simulink model "gps_tracking_onlydll_hwc_2"  (R2018a)
settings: Solver=VariableStepAuto  StartTime=0.0  StopTime=10*16368/16367600  RelTol=1e-3
libraries: xbsIndex_r4 x101, dspsrcs4 x1
settings Model: Creator=zhati  LastModifiedBy=Doc_v
settings CodeAppCC: StateflowObjectComments=on
settings SimscapeCC: SimscapeNormalizeSystem=off

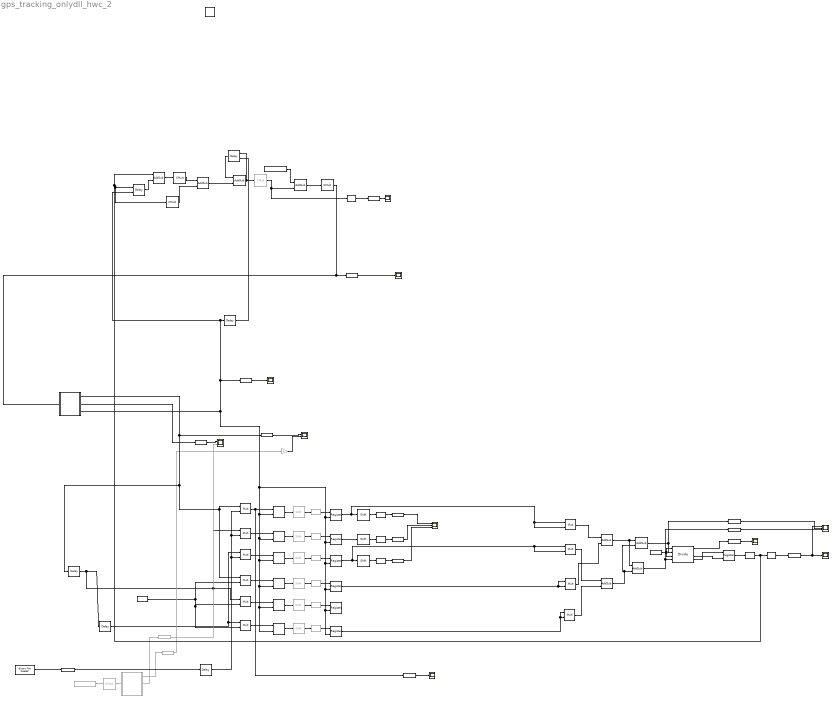
== system gps_tracking_onlydll_hwc_2 ==
  note: Subsystem1
  note: Subsystem
  note: Subsystem1
  " I_P_Out" : xbsIndex_r4/Gateway Out  inherit_from_input=on  hdl_port=on  rows=1  columns=1  UseAsDAC=off  DACChannel='1'  interface=None  automatic_assignment=on  address_offset=hex2dec('00')  intf_name=''  intf_description=''  timing_constraint=None  locs_specified=off  LOCs={}  io_standard={}  block_type=gatewayout
  " System Generator" : xbsIndex_r4/ System Generator  Tag=genX  xilinxfamily=kintex7  part=xc7k325t  speed=-2  package=ffg900  synthesis_tool=Vivado  clock_wrapper=Clock Enables  directory=./gps_tracking_onlydll_hwc2  proj_type=Vivado  Synth_file=Vivado Synthesis Defaults  Impl_file=Vivado Implementation Defaults  testbench=on  simulink_period=1/16367600  sysclk_period=10  dcm_input_clock_period=10  incr_netlist=off  trim_vbits=Everywhere in SubSystem  dbl_ovrd=According to Block Masks  core_generation=According to Block Masks  run_coregen=off  deprecated_control=off  eval_field=0  block_type=sysgen
  Accumulator{,1..5} (6 alike) : xbsIndex_r4/Accumulator  operation=Add  n_bits=20  overflow=Wrap  scale=1  rst=on  hasbypass=off  infoeditControl=reset for floating point data type must be asserted for a minimum of 2 cycles  en=off  latency=1  msb_inp=100  msb=100  lsb=-100  use_behavioral_HDL=on  implementation=Fabric  dbl_ovrd=off  block_type=accum
  AddSub10 : xbsIndex_r4/AddSub  mode=Addition  use_carryin=off  use_carryout=off  en=off  latency=1  precision=User Defined  arith_type="Signed  (2's comp)"  n_bits=35  bin_pt=0  quantization=Truncate  overflow=Flag as error  use_behavioral_HDL=off  hw_selection=Fabric  pipelined=off  dbl_ovrd=off  block_type=addsub
  AddSub11 : xbsIndex_r4/AddSub  mode=Subtraction  use_carryin=off  use_carryout=off  en=off  latency=1  precision=User Defined  arith_type="Signed  (2's comp)"  n_bits=35  bin_pt=0  quantization=Truncate  overflow=Flag as error  use_behavioral_HDL=off  hw_selection=Fabric  pipelined=off  dbl_ovrd=off  block_type=addsub
  AddSub{5,7,9,12} (4 alike) : xbsIndex_r4/AddSub  mode=Addition  use_carryin=off  use_carryout=off  en=off  latency=1  precision=Full  arith_type="Signed  (2's comp)"  n_bits=16  bin_pt=15  quantization=Truncate  overflow=Wrap  use_behavioral_HDL=off  hw_selection=Fabric  pipelined=off  dbl_ovrd=off  block_type=addsub
  AddSub2 : xbsIndex_r4/AddSub  mode=Subtraction  use_carryin=off  use_carryout=off  en=off  latency=1  precision=Full  arith_type="Signed  (2's comp)"  n_bits=16  bin_pt=15  quantization=Truncate  overflow=Wrap  use_behavioral_HDL=off  hw_selection=Fabric  pipelined=off  dbl_ovrd=off  block_type=addsub
  AddSub6 : xbsIndex_r4/AddSub  mode=Addition  use_carryin=off  use_carryout=off  en=off  latency=1  precision=User Defined  arith_type="Signed  (2's comp)"  n_bits=32  bin_pt=15  quantization=Truncate  overflow=Flag as error  use_behavioral_HDL=off  hw_selection=Fabric  pipelined=off  dbl_ovrd=off  block_type=addsub
  Binary File Reader : dspsrcs4/Binary File Reader  Filename=E:\sysgen_workspace\myGNSSdata_BB.bin  HeaderStructure=struct([])  DataType=int8  SamplesPerFrame=1  IsDataComplex=off  NumChannels=1  OutputEOF=off  SampleTime=1/16367600  SimulateUsing=Code generation
      settings: SourceProductName=DSP System Toolbox  SourceProductBaseCode=DS
  Constant : xbsIndex_r4/Constant  const=0  gui_display_data_type=Fixed-point  arith_type=Signed (2's comp)  n_bits=4  bin_pt=3  preci_type=Single  exp_width=8  frac_width=24  explicit_period=on  period=1/16367600  equ=P=C  opselect=C  inp2=PCIN>>17  opr=+  inp1=P  carry=CIN  dbl_ovrd=off  block_type=constant
  Constant1 : xbsIndex_r4/Constant  const=1.0  gui_display_data_type=Boolean  arith_type=Boolean  n_bits=16  bin_pt=14  preci_type=Single  exp_width=8  frac_width=24  explicit_period=off  period=1  equ=P=C  opselect=C  inp2=PCIN>>17  opr=+  inp1=P  carry=CIN  dbl_ovrd=off  block_type=constant
  Convert : xbsIndex_r4/Convert  gui_display_data_type=Fixed-point  arith_type="Signed  (2's comp)"  n_bits=16  bin_pt=0  float_type=Single  exp_bits=8  fraction_bits=24  quantization=Truncate  overflow=Saturate  en=off  latency=1  pipeline=off  dbl_ovrd=off  block_type=convert
  Convert{1..6} (6 alike) : xbsIndex_r4/Convert  Commented=through  gui_display_data_type=Fixed-point  arith_type="Signed  (2's comp)"  n_bits=26  bin_pt=26  float_type=Single  exp_bits=8  fraction_bits=24  quantization=Truncate  overflow=Flag as error  en=off  latency=1  pipeline=off  dbl_ovrd=off  block_type=convert
  Convert10 : xbsIndex_r4/Convert  gui_display_data_type=Fixed-point  arith_type="Signed  (2's comp)"  n_bits=8  bin_pt=4  float_type=Single  exp_bits=8  fraction_bits=24  quantization=Truncate  overflow=Saturate  en=off  latency=1  pipeline=off  dbl_ovrd=off  block_type=convert
  Convert11 : xbsIndex_r4/Convert  gui_display_data_type=Fixed-point  arith_type="Signed  (2's comp)"  n_bits=8  bin_pt=7  float_type=Single  exp_bits=8  fraction_bits=24  quantization=Truncate  overflow=Saturate  en=off  latency=1  pipeline=off  dbl_ovrd=off  block_type=convert
  Convert7 : xbsIndex_r4/Convert  gui_display_data_type=Fixed-point  arith_type="Signed  (2's comp)"  n_bits=8  bin_pt=0  float_type=Single  exp_bits=8  fraction_bits=24  quantization=Truncate  overflow=Saturate  en=off  latency=1  pipeline=off  dbl_ovrd=off  block_type=convert
  Convert8 : xbsIndex_r4/Convert  gui_display_data_type=Fixed-point  arith_type="Signed  (2's comp)"  n_bits=8  bin_pt=0  float_type=Single  exp_bits=8  fraction_bits=24  quantization=Truncate  overflow=Saturate  en=off  latency=1  pipeline=off  dbl_ovrd=off  block_type=convert
  Convert9 : xbsIndex_r4/Convert  gui_display_data_type=Fixed-point  arith_type="Signed  (2's comp)"  n_bits=16  bin_pt=14  float_type=Single  exp_bits=8  fraction_bits=24  quantization=Truncate  overflow=Saturate  en=off  latency=1  pipeline=off  dbl_ovrd=off  block_type=convert
  D1 : xbsIndex_r4/CMult  const=5.297297  gui_display_data_type=Fixed-point  const_n_bits=20  const_bin_pt=15  float_type=Single  exp_bits=8  fraction_bits=24  en=off  latency=1  precision=Full  arith_type="Signed  (2's comp)"  n_bits=16  bin_pt=14  quantization=Truncate  overflow=Wrap  use_behavioral_HDL=off  mem_type=Distributed RAM  pipeline=off  dbl_ovrd=off  block_type=cmult
  D2 : xbsIndex_r4/CMult  const=1/16367600  gui_display_data_type=Fixed-point  const_n_bits=48  const_bin_pt=48  float_type=Single  exp_bits=8  fraction_bits=24  en=off  latency=1  precision=User Defined  arith_type="Signed  (2's comp)"  n_bits=32  bin_pt=32  quantization=Truncate  overflow=Flag as error  use_behavioral_HDL=off  mem_type=Distributed RAM  pipeline=off  dbl_ovrd=off  block_type=cmult
  D3 : xbsIndex_r4/CMult  Commented=through  const=10  gui_display_data_type=Fixed-point  const_n_bits=8  const_bin_pt=0  float_type=Single  exp_bits=8  fraction_bits=24  en=off  latency=1  precision=User Defined  arith_type="Signed  (2's comp)"  n_bits=26  bin_pt=16  quantization=Truncate  overflow=Flag as error  use_behavioral_HDL=off  mem_type=Distributed RAM  pipeline=off  dbl_ovrd=off  block_type=cmult
  D4 : xbsIndex_r4/CMult  Commented=on  const=1/16367600  gui_display_data_type=Fixed-point  const_n_bits=48  const_bin_pt=48  float_type=Single  exp_bits=8  fraction_bits=24  en=off  latency=1  precision=User Defined  arith_type="Signed  (2's comp)"  n_bits=26  bin_pt=22  quantization=Truncate  overflow=Flag as error  use_behavioral_HDL=off  mem_type=Distributed RAM  pipeline=off  dbl_ovrd=off  block_type=cmult
  DLLFilteredOut : xbsIndex_r4/Gateway Out  inherit_from_input=off  hdl_port=on  rows=1  columns=1  UseAsDAC=off  DACChannel='1'  interface=None  automatic_assignment=on  address_offset=hex2dec('00')  intf_name=''  intf_description=''  timing_constraint=None  locs_specified=off  LOCs={}  io_standard={}  block_type=gatewayout
  DLLRawDiscriminatorOut : xbsIndex_r4/Gateway Out  inherit_from_input=on  hdl_port=on  rows=1  columns=1  UseAsDAC=off  DACChannel='1'  interface=None  automatic_assignment=on  address_offset=hex2dec('00')  intf_name=''  intf_description=''  timing_constraint=None  locs_specified=off  LOCs={}  io_standard={}  block_type=gatewayout
  Delay2 : xbsIndex_r4/Delay  rst=off  infoeditControl=Selection of Reset will increase slice count due to use of real FFs and instead of SRLs  en=off  latency=28  reg_retiming=off  dbl_ovrd=off  block_type=delay
  Delay4 : xbsIndex_r4/Delay  rst=off  infoeditControl=Selection of Reset will increase slice count due to use of real FFs and instead of SRLs  en=off  latency=8  reg_retiming=off  dbl_ovrd=off  block_type=delay
  Delay5 : xbsIndex_r4/Delay  rst=off  infoeditControl=Selection of Reset will increase slice count due to use of real FFs and instead of SRLs  en=on  latency=1  reg_retiming=off  dbl_ovrd=off  block_type=delay
  Delay6 : xbsIndex_r4/Delay  rst=off  infoeditControl=Selection of Reset will increase slice count due to use of real FFs and instead of SRLs  en=off  latency=8  reg_retiming=off  dbl_ovrd=off  block_type=delay
  Delay7 : xbsIndex_r4/Delay  rst=off  infoeditControl=Selection of Reset will increase slice count due to use of real FFs and instead of SRLs  en=on  latency=1  reg_retiming=off  dbl_ovrd=off  block_type=delay
  Delay8 : xbsIndex_r4/Delay  rst=off  infoeditControl=Selection of Reset will increase slice count due to use of real FFs and instead of SRLs  en=off  latency=3  reg_retiming=off  dbl_ovrd=off  block_type=delay
  Divide : xbsIndex_r4/Divide  flow_control=Blocking  axi_optimize_goal=Resources  algorithm_type=High_Radix  infoedit1=Specify output fraction-width for Fixed-point division.  fractional_width=14  infoedit2=Specify latency for Floating-point division.  latency=1  rate=1  has_a_tlast=off  has_a_tuser=off  has_b_tlast=off  has_b_tuser=off  en=off  has_result_tready=off  result_tlast_behv=Pass_A_TLAST  has_underflow=off  has_overflow=off  has_invalid_op=off  has_divide_by_zero=off  fpo_op_type=mergeddivide  block_type=divide
      settings: infoedit=Blocking: Wait for data on all inputs, allow back-pressure.<br>NonBlocking: operate every cycle in which all inputs are valid, no back-pressure.
  E_I : xbsIndex_r4/Mult  precision=Full  arith_type="Signed  (2's comp)"  n_bits=16  bin_pt=14  quantization=Truncate  overflow=Wrap  en=off  latency=1  use_behavioral_HDL=off  opt=Speed  use_embedded=on  optimum_pipeline=off  pipeline=on  dbl_ovrd=off  use_rpm=on  placement_style=Triangular  block_type=mult
  E_Q : xbsIndex_r4/Mult  precision=Full  arith_type="Signed  (2's comp)"  n_bits=16  bin_pt=14  quantization=Truncate  overflow=Wrap  en=off  latency=1  use_behavioral_HDL=off  opt=Speed  use_embedded=on  optimum_pipeline=off  pipeline=on  dbl_ovrd=off  use_rpm=on  placement_style=Triangular  block_type=mult
  E_mult : xbsIndex_r4/Mult  precision=Full  arith_type="Signed  (2's comp)"  n_bits=16  bin_pt=14  quantization=Truncate  overflow=Wrap  en=off  latency=1  use_behavioral_HDL=off  opt=Speed  use_embedded=on  optimum_pipeline=off  pipeline=on  dbl_ovrd=off  use_rpm=on  placement_style=Triangular  block_type=mult
  E_mult1 : xbsIndex_r4/Mult  precision=Full  arith_type="Signed  (2's comp)"  n_bits=16  bin_pt=14  quantization=Truncate  overflow=Wrap  en=off  latency=1  use_behavioral_HDL=off  opt=Speed  use_embedded=on  optimum_pipeline=off  pipeline=on  dbl_ovrd=off  use_rpm=on  placement_style=Triangular  block_type=mult
  F1 : xbsIndex_r4/Constant  const=1023000  gui_display_data_type=Fixed-point  arith_type=Signed (2's comp)  n_bits=32  bin_pt=8  preci_type=Single  exp_width=8  frac_width=24  explicit_period=on  period=1/16367600  equ=P=C  opselect=C  inp2=PCIN>>17  opr=+  inp1=P  carry=CIN  dbl_ovrd=off  block_type=constant
  F2 : xbsIndex_r4/Constant  Commented=on  const=1023000  gui_display_data_type=Fixed-point  arith_type=Signed (2's comp)  n_bits=32  bin_pt=8  preci_type=Single  exp_width=8  frac_width=24  explicit_period=on  period=1/16367600  equ=P=C  opselect=C  inp2=PCIN>>17  opr=+  inp1=P  carry=CIN  dbl_ovrd=off  block_type=constant
  Gain1 : Gain  Commented=through  Gain=5
  Gateway Out{3,6..8} (4 alike) : xbsIndex_r4/Gateway Out  inherit_from_input=off  hdl_port=off  rows=1  columns=1  UseAsDAC=off  DACChannel='1'  interface=None  automatic_assignment=on  address_offset=hex2dec('00')  intf_name=''  intf_description=''  timing_constraint=None  locs_specified=off  LOCs={}  io_standard={}  block_type=gatewayout
  Gateway Out4 : xbsIndex_r4/Gateway Out  Commented=on  inherit_from_input=off  hdl_port=off  rows=1  columns=1  UseAsDAC=off  DACChannel='1'  interface=None  automatic_assignment=on  address_offset=hex2dec('00')  intf_name=''  intf_description=''  timing_constraint=None  locs_specified=off  LOCs={}  io_standard={}  block_type=gatewayout
  Gateway Out_A : xbsIndex_r4/Gateway Out  inherit_from_input=off  hdl_port=off  rows=1  columns=1  UseAsDAC=off  DACChannel='1'  interface=None  automatic_assignment=on  address_offset=hex2dec('00')  intf_name=''  intf_description=''  timing_constraint=None  locs_specified=off  LOCs={}  io_standard={}  block_type=gatewayout
  Gateway Out_B : xbsIndex_r4/Gateway Out  inherit_from_input=off  hdl_port=off  rows=1  columns=1  UseAsDAC=off  DACChannel='1'  interface=None  automatic_assignment=on  address_offset=hex2dec('00')  intf_name=''  intf_description=''  timing_constraint=None  locs_specified=off  LOCs={}  io_standard={}  block_type=gatewayout
  I2 : xbsIndex_r4/CMult  const=0.014317  gui_display_data_type=Fixed-point  const_n_bits=20  const_bin_pt=15  float_type=Single  exp_bits=8  fraction_bits=24  en=off  latency=2  precision=Full  arith_type="Signed  (2's comp)"  n_bits=16  bin_pt=14  quantization=Truncate  overflow=Wrap  use_behavioral_HDL=off  mem_type=Distributed RAM  pipeline=off  dbl_ovrd=off  block_type=cmult
  IF In : xbsIndex_r4/Gateway In  gui_display_data_type=Fixed-point  arith_type="Signed  (2's comp)"  n_bits=3  bin_pt=0  preci_type=Single  exp_width=8  frac_width=24  rows=1  columns=1  quantization="Round  (unbiased: +/- Inf)"  overflow=Flag as error  period=1/16367600  UseAsADC=off  ADCChannel='1'  interface=None  automatic_assignment=on  address_offset=hex2dec('00')  intf_name=''  intf_description=''  default_value=0  timing_constraint=None  locs_specified=off  LOCs={}  io_standard={}  inherit_from_input=off  hdl_port=on  dbl_ovrd=off  block_type=gatewayin
  IF Out : xbsIndex_r4/Gateway Out  Commented=on  inherit_from_input=off  hdl_port=off  rows=1  columns=1  UseAsDAC=off  DACChannel='1'  interface=None  automatic_assignment=on  address_offset=hex2dec('00')  intf_name=''  intf_description=''  timing_constraint=None  locs_specified=off  LOCs={}  io_standard={}  block_type=gatewayout
  I_E_Out : xbsIndex_r4/Gateway Out  inherit_from_input=on  hdl_port=on  rows=1  columns=1  UseAsDAC=off  DACChannel='1'  interface=None  automatic_assignment=on  address_offset=hex2dec('00')  intf_name=''  intf_description=''  timing_constraint=None  locs_specified=off  LOCs={}  io_standard={}  block_type=gatewayout
  I_L_Out : xbsIndex_r4/Gateway Out  inherit_from_input=on  hdl_port=on  rows=1  columns=1  UseAsDAC=off  DACChannel='1'  interface=None  automatic_assignment=on  address_offset=hex2dec('00')  intf_name=''  intf_description=''  timing_constraint=None  locs_specified=off  LOCs={}  io_standard={}  block_type=gatewayout
  L_I : xbsIndex_r4/Mult  precision=Full  arith_type="Signed  (2's comp)"  n_bits=16  bin_pt=14  quantization=Truncate  overflow=Wrap  en=off  latency=1  use_behavioral_HDL=off  opt=Speed  use_embedded=on  optimum_pipeline=off  pipeline=on  dbl_ovrd=off  use_rpm=on  placement_style=Triangular  block_type=mult
  L_Q : xbsIndex_r4/Mult  precision=Full  arith_type="Signed  (2's comp)"  n_bits=16  bin_pt=14  quantization=Truncate  overflow=Wrap  en=off  latency=1  use_behavioral_HDL=off  opt=Speed  use_embedded=on  optimum_pipeline=off  pipeline=on  dbl_ovrd=off  use_rpm=on  placement_style=Triangular  block_type=mult
  Multi Out : xbsIndex_r4/Gateway Out  inherit_from_input=off  hdl_port=off  rows=1  columns=1  UseAsDAC=off  DACChannel='1'  interface=None  automatic_assignment=on  address_offset=hex2dec('00')  intf_name=''  intf_description=''  timing_constraint=None  locs_specified=off  LOCs={}  io_standard={}  block_type=gatewayout
  PNGen Out : xbsIndex_r4/Gateway Out  inherit_from_input=off  hdl_port=off  rows=1  columns=1  UseAsDAC=off  DACChannel='1'  interface=None  automatic_assignment=on  address_offset=hex2dec('00')  intf_name=''  intf_description=''  timing_constraint=None  locs_specified=off  LOCs={}  io_standard={}  block_type=gatewayout
  Register{1..7} (7 alike) : xbsIndex_r4/Register  init=0  rst=off  en=on  dbl_ovrd=off  block_type=register
  Scope : Scope
  Scope1 : Scope
  Scope2_en : Scope
  Scope6 : Scope  NumInputPorts=2
  Scope_CACode : Scope  NumInputPorts=2
  Scope_CodeFreq : Scope
  Scope_DLLDiscriminator : Scope  NumInputPorts=3
  Scope_I_ELP : Scope  NumInputPorts=3
  Scope_MultiResult : Scope
  Shift{,1..5} (6 alike) : xbsIndex_r4/Shift  Commented=through  shift_dir=Right  shift_bits=16  en=off  latency=1  precision=Full  arith_type="Signed  (2's comp)"  n_bits=16  bin_pt=14  quantization=Truncate  overflow=Wrap  dbl_ovrd=off  block_type=shift
  Shift6 : xbsIndex_r4/Shift  shift_dir=Right  shift_bits=8  en=off  latency=1  precision=Full  arith_type="Signed  (2's comp)"  n_bits=16  bin_pt=14  quantization=Truncate  overflow=Wrap  dbl_ovrd=off  block_type=shift
  Shift7 : xbsIndex_r4/Shift  shift_dir=Right  shift_bits=8  en=off  latency=1  precision=Full  arith_type="Signed  (2's comp)"  n_bits=16  bin_pt=14  quantization=Truncate  overflow=Wrap  dbl_ovrd=off  block_type=shift
  Shift8 : xbsIndex_r4/Shift  shift_dir=Right  shift_bits=8  en=off  latency=1  precision=Full  arith_type="Signed  (2's comp)"  n_bits=16  bin_pt=14  quantization=Truncate  overflow=Wrap  dbl_ovrd=off  block_type=shift
  Subsystem : Subsystem
  Subsystem1 : Subsystem  Commented=on
  l_mult : xbsIndex_r4/Mult  precision=Full  arith_type="Signed  (2's comp)"  n_bits=16  bin_pt=14  quantization=Truncate  overflow=Wrap  en=off  latency=1  use_behavioral_HDL=off  opt=Speed  use_embedded=on  optimum_pipeline=off  pipeline=on  dbl_ovrd=off  use_rpm=on  placement_style=Triangular  block_type=mult
  l_mult1 : xbsIndex_r4/Mult  precision=Full  arith_type="Signed  (2's comp)"  n_bits=16  bin_pt=14  quantization=Truncate  overflow=Wrap  en=off  latency=1  use_behavioral_HDL=off  opt=Speed  use_embedded=on  optimum_pipeline=off  pipeline=on  dbl_ovrd=off  use_rpm=on  placement_style=Triangular  block_type=mult
  p_mult : xbsIndex_r4/Mult  precision=Full  arith_type="Signed  (2's comp)"  n_bits=16  bin_pt=14  quantization=Truncate  overflow=Wrap  en=off  latency=1  use_behavioral_HDL=off  opt=Speed  use_embedded=on  optimum_pipeline=off  pipeline=on  dbl_ovrd=off  use_rpm=on  placement_style=Triangular  block_type=mult
  p_mult1 : xbsIndex_r4/Mult  precision=Full  arith_type="Signed  (2's comp)"  n_bits=16  bin_pt=14  quantization=Truncate  overflow=Wrap  en=off  latency=1  use_behavioral_HDL=off  opt=Speed  use_embedded=on  optimum_pipeline=off  pipeline=on  dbl_ovrd=off  use_rpm=on  placement_style=Triangular  block_type=mult
  scope_codenco : Scope
  wires:
  Binary File Reader/1 -> IF In/1
  Gateway Out8/1 -> Scope6/1
  I_L_Out/1 -> Scope_I_ELP/3
  " I_P_Out"/1 -> Scope_I_ELP/2
  Constant/1 -> l_mult/2, p_mult/2, E_mult/2
  Delay4/1 -> p_mult1/1, p_mult/1, Delay6/1
  Convert2/1 -> Register2/1
  Accumulator1/1 -> Shift/1
  E_mult/1 -> Accumulator3/1
  l_mult1/1 -> Accumulator2/1
  l_mult/1 -> Accumulator5/1
  E_mult1/1 -> Multi Out/1, Accumulator1/1
  Delay6/1 -> l_mult/1, l_mult1/1
  p_mult1/1 -> Accumulator/1
  p_mult/1 -> Accumulator4/1
  Multi Out/1 -> Scope_MultiResult/1
  PNGen Out/1 -> Scope_CACode/1
  Gain1/1 -> Scope_CACode/2
  I_E_Out/1 -> Scope_I_ELP/1
  Shift/1 -> Convert2/1
  Shift1/1 -> Convert1/1
  Convert1/1 -> Register3/1
  Accumulator/1 -> Shift1/1
  Shift2/1 -> Convert3/1
  Accumulator2/1 -> Shift2/1
  Convert3/1 -> Register4/1
  Convert4/1 -> Register5/1
  Accumulator3/1 -> Shift3/1
  Shift3/1 -> Convert4/1
  Shift4/1 -> Convert5/1
  Accumulator4/1 -> Shift4/1
  Convert5/1 -> Register6/1
  Convert6/1 -> Register7/1
  Accumulator5/1 -> Shift5/1
  Shift5/1 -> Convert6/1
  DLLRawDiscriminatorOut/1 -> Scope_DLLDiscriminator/1, Scope1/1
  Gateway Out_A/1 -> Scope_DLLDiscriminator/2
  Gateway Out_B/1 -> Scope_DLLDiscriminator/3
  Gateway Out6/1 -> Scope_CodeFreq/1
  AddSub11/1 -> Divide/2, Gateway Out_A/1
  AddSub10/1 -> Divide/4, Gateway Out_B/1
  AddSub9/1 -> AddSub11/1, AddSub10/1
  E_Q/1 -> AddSub9/2
  Register7/1 -> L_Q/1, L_Q/2
  Register5/1 -> E_Q/1, E_Q/2
  AddSub12/1 -> AddSub10/2, AddSub11/2
  L_I/1 -> AddSub12/1
  E_I/1 -> AddSub9/1
  L_Q/1 -> AddSub12/2
  Register4/1 -> Shift8/1, L_I/2, L_I/1
  Constant1/1 -> Divide/1, Divide/3
  Gateway Out3/1 -> Scope/1
  Divide/3 -> Register1/2
  Divide/4 -> Register1/1
  Divide/1 -> Gateway Out3/1
  IF Out/1 -> Gain1/1
  Gateway Out4/1 -> Scope6/2
  Delay2/1 -> l_mult1/2, E_mult1/2, p_mult1/2
  DLLFilteredOut/1 -> scope_codenco/1
  Gateway Out7/1 -> Scope2_en/1
  Subsystem/1(ROM Out) -> PNGen Out/1, Delay4/1, E_mult/1, E_mult1/1
  Subsystem/2(Addr Out) -> Gateway Out8/1
  D2/1 -> Gateway Out6/1, Subsystem/1(CodeFreqIn)
  D3/1 -> Convert10/1, AddSub7/2
  AddSub6/1 -> D3/1, Delay7/1
  Register1/1 -> Convert9/1
  Subsystem/3(EN Out) -> Gateway Out7/1, Delay5/2, Delay8/1, Register3/2, Register4/2, Register5/2, Register7/2, Register6/2, Register2/2, Accumulator5/2, Accumulator4/2, Accumulator3/2, Accumulator2/2, Accumulator/2, Accumulator1/2
  AddSub7/1 -> D2/1
  I2/1 -> AddSub5/2
  AddSub2/1 -> D1/1
  F1/1 -> AddSub7/1
  Delay7/1 -> AddSub6/1
  Delay8/1 -> Delay7/2
  AddSub5/1 -> AddSub6/2
  Delay5/1 -> AddSub2/2
  D1/1 -> AddSub5/1
  Subsystem1/2(Addr Out) -> Gateway Out4/1
  Subsystem1/1(ROM Out) -> IF Out/1
  D4/1 -> Subsystem1/1(CodeFreqIn)
  F2/1 -> D4/1
  IF In/1 -> Delay2/1
  Convert/1 -> I_L_Out/1
  Convert7/1 -> " I_P_Out"/1
  Convert8/1 -> I_E_Out/1
  Register2/1 -> Shift6/1, E_I/2, E_I/1
  Register3/1 -> Shift7/1
  Convert9/1 -> Convert11/1, Delay5/1, I2/1, AddSub2/1
  Convert10/1 -> DLLFilteredOut/1
  Convert11/1 -> DLLRawDiscriminatorOut/1
  Shift6/1 -> Convert8/1
  Shift7/1 -> Convert7/1
  Shift8/1 -> Convert/1

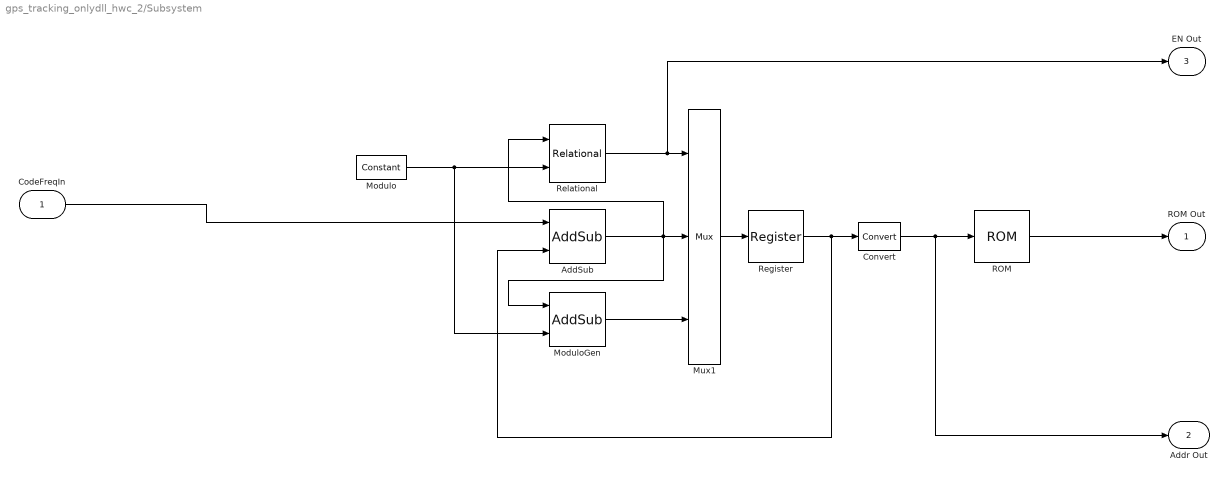
== system gps_tracking_onlydll_hwc_2/Subsystem ==
  CodeFreqIn : Inport
  AddSub : xbsIndex_r4/AddSub  mode=Addition  use_carryin=off  use_carryout=off  en=off  latency=0  precision=User Defined  arith_type=Unsigned  n_bits=42  bin_pt=32  quantization=Truncate  overflow=Flag as error  use_behavioral_HDL=off  hw_selection=Fabric  pipelined=off  dbl_ovrd=off  block_type=addsub
  Convert : xbsIndex_r4/Convert  gui_display_data_type=Fixed-point  arith_type=Unsigned  n_bits=10  bin_pt=0  float_type=Single  exp_bits=8  fraction_bits=24  quantization=Truncate  overflow=Wrap  en=off  latency=1  pipeline=off  dbl_ovrd=off  block_type=convert
  Modulo : xbsIndex_r4/Constant  const=1023-2e-32  gui_display_data_type=Fixed-point  arith_type=Unsigned  n_bits=42  bin_pt=32  preci_type=Single  exp_width=8  frac_width=24  explicit_period=on  period=1/16367600  equ=P=C  opselect=C  inp2=PCIN>>17  opr=+  inp1=P  carry=CIN  dbl_ovrd=off  block_type=constant
  ModuloGen : xbsIndex_r4/AddSub  mode=Subtraction  use_carryin=off  use_carryout=off  en=off  latency=0  precision=User Defined  arith_type=Unsigned  n_bits=42  bin_pt=32  quantization=Truncate  overflow=Wrap  use_behavioral_HDL=off  hw_selection=Fabric  pipelined=off  dbl_ovrd=off  block_type=addsub
  Mux1 : xbsIndex_r4/Mux  inputs=2  en=off  latency=0  precision=Full  arith_type=Unsigned  n_bits=16  bin_pt=14  quantization=Truncate  overflow=Wrap  dbl_ovrd=off  block_type=mux
  ROM : xbsIndex_r4/ROM  depth=1023  initVector=[1,-1,-1,1,-1,1,1,-1,1,1,-1,-1,-1,1,-1,-1,-1,1,1,-1,1,1,-1,-1,-1,1,-1,1,-1,1,1,1,-1,-1,-1,1,1,1,1,-1,1,-1,1,-1,1,1,1,-1,1,1,1,1,1,-1,-1,1,1,-1,1,1,1,1,1,-1,1,-1,1,-1,-1,-1,1,1,1,1,1,-1,1,1,1,-1,-1,1,-1,-1,-1,1,-1,1,1,-1,-1,1,-1,-1,1,1,1,-1,1,-1,1,1,1,1,-1,1,1,-1,-1,1,-1,-1,1,-1,-1,-1,-1,1,1,-1,-1,-1,-1,-1,-1,-1,-1,1,1,1,-1,-1,-1,-1,-1,-1,1,1,1,-1,-1,1,1,1,1,-1,1,1,1,1,-1,1,-1,-1,1,-1,-1,1,1,-1,1,1,-1,1,1,1,-1,1,1,-1,-1,1,-1,1,1,-1,1,1,1,1,-1,-1,1,1,1,1,-1,1,1,1,-1,-1,1,-1,-1,1,1,-1,1,1,-1,1,1,-1,-1,1,1,1,-1,-1,-1,1,-1,-1,-1,-1,-1,-1,-1,1,-1,-1,1,-1,-1,1,-1,1,-1,-1,-1,1,1,1,1,1,1,1,1,-1,-1,-1,-1,1,1,1,-1,-1,1,-1,1,1,-1,1,1,-1,1,-1,-1,-1,1,1,1,-1,-1,1,1,1,-1,1,1,1,-1,1,-1,-1,-1,1,1,-1,1,1,1,-1,-1,-1,1,-1,1,-1,-1,-1,-1,-1,-1,1,-1,1,1,-1,1,-1,-1,-1,-1,1,-1,-1,1,1,-1,1,-1,1,1,1,1,-1,-1,-1,1,1,1,1,1,1,-1,-1,-1,1,-1,-1,1,1,-1,-1,1,1,-1,-1,-1,-1,-1,-1,-1,1,-1,1,1,1,1,1,1,1,1,1,-1,-1,1,1,-1,-1,-1,1,-1,1,1,-1,-1,1,-1,1,1,1,1,1,-1,-1,1,-1,-1,1,-1,-1,1,-1,1,-1,1,-1,-1,1,1,1,1,1,-1,1,-1,1,-1,1,1,-1,-1,1,-1,1,1,-1,1,-1,-1,1,-1,-1,1,1,-1,-1,-1,-1,-1,-1,-1,1,1,-1,-1,-1,-1,-1,-1,1,-1,1,1,1,-1,1,1,-1,1,-1,-1,-1,-1,1,-1,-1,-1,1,1,1,1,-1,1,1,-1,1,1,-1,1,-1,-1,-1,1,1,-1,1,1,-1,-1,-1,-1,1,1,1,-1,1,-1,-1,1,-1,-1,-1,-1,1,1,1,-1,-1,-1,-1,1,1,-1,-1,1,1,-1,-1,-1,1,-1,-1,-1,-1,1,-1,1,-1,-1,1,-1,-1,-1,-1,-1,1,-1,-1,1,1,-1,1,-1,-1,1,-1,1,-1,-1,-1,1,-1,1,1,-1,1,1,-1,1,-1,1,-1,1,-1,1,-1,1,-1,-1,-1,1,1,1,-1,1,-1,1,1,1,-1,1,1,1,-1,-1,-1,-1,1,-1,1,1,-1,-1,1,-1,1,-1,1,-1,1,1,1,1,1,1,1,1,1,-1,-1,-1,1,-1,-1,1,1,1,1,1,1,-1,-1,1,-1,-1,1,-1,-1,1,-1,-1,-1,-1,-1,-1,-1,1,1,-1,1,1,-1,1,1,1,-1,-1,-1,-1,1,-1,1,-1,1,1,1,1,-1,1,1,-1,1,1,1,1,1,-1,-1,-1,-1,1,-1,-1,1,1,-1,-1,1,1,1,-1,1,1,1,1,-1,-1,-1,1,1,1,1,1,-1,1,-1,1,-1,1,-1,-1,1,1,1,-1,1,-1,-1,1,1,1,-1,1,-1,-1,-1,-1,-1,1,1,1,-1,1,-1,-1,1,1,1,-1,-1,1,1,1,1,1,-1,1,-1,-1,-1,1,1,1,-1,1,1,1,1,-1,-1,-1,1,1,1,-1,-1,-1,1,-1,-1,1,-1,-1,-1,-1,1,-1,1,1,1,-1,1,1,1,-1,1,1,-1,-1,1,-1,-1,1,-1,-1,1,1,-1,-1,1,1,-1,-1,-1,-1,-1,-1,1,1,-1,1,1,-1,1,-1,-1,-1,1,1,1,-1,1,-1,1,1,1,-1,1,-1,1,-1,-1,-1,1,1,1,-1,-1,-1,-1,-1,-1,1,1,-1,1,-1,-1,-1,-1,1,1,1,-1,-1,-1,-1,1,-1,1,-1,1,-1,-1,-1,-1,-1,-1,1,1,1,1,1,1,-1,-1,1,1,-1,1,1,1,1,-1,1,1,-1,1,-1,1,-1,1,-1,1,-1,-1,1,-1,-1,-1,1,1,-1,-1,-1,-1,-1,-1,-1,-1,1,1,-1,-1,1,-1,-1,1,-1,1,-1,1,1,1,-1,1,-1,-1,1,1,1,1,1,-1,-1,1,-1,-1,1,1,-1,-1,1,1,-1,1,-1,-1,1,-1,1,-1,-1,-1,1,1,-1,1,-1,1,-1,1,-1,-1,1,1,1,1,-1,-1,-1,-1,-1,-1,1,1,1,1,1,-1,-1,1,-1,-1,-1,1,1,1,-1,1,-1,1,-1,1,-1,1,1,-1,-1,-1,1,-1,1,1,1,-1,-1,1,1,1,1,-1,1,-1,1,1,-1,1,-1,1,-1,-1,1,1,-1,1,-1,-1,-1,-1,-1,1,-1,-1,1,1,-1,1,-1,1,-1,-1,1,1,1,-1,-1,1,-1]  distributed_mem=Block RAM  rst=off  init_reg=0  en=off  latency=1  gui_display_data_type=Fixed-point  arith_type="Signed  (2's comp)"  n_bits=2  bin_pt=0  preci_type=Single  exp_width=8  frac_width=24  optimize=Area  use_rpm=on  dbl_ovrd=off  block_type=sprom
  Register : xbsIndex_r4/Register  init=0  rst=off  en=off  dbl_ovrd=off  block_type=register
  Relational : xbsIndex_r4/Relational  mode=a>=b  op_type=Bool  en=off  latency=0  dbl_ovrd=off  block_type=relational
  ROM Out : Outport
  Addr Out : Outport  Port=2
  EN Out : Outport  Port=3
  wires:
  Relational/1 -> EN Out/1, Mux1/1
  Convert/1 -> ROM/1, Addr Out/1
  ROM/1 -> ROM Out/1
  CodeFreqIn/1 -> AddSub/1
  Mux1/1 -> Register/1
  AddSub/1 -> ModuloGen/1, Relational/1, Mux1/2
  ModuloGen/1 -> Mux1/3
  Modulo/1 -> ModuloGen/2, Relational/2
  Register/1 -> Convert/1, AddSub/2

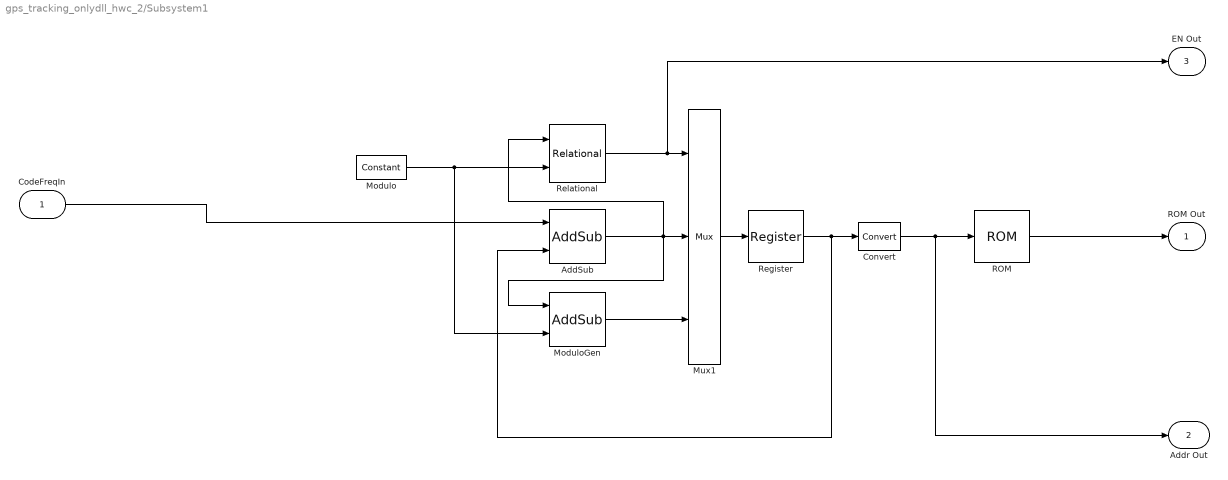
== system gps_tracking_onlydll_hwc_2/Subsystem1 ==
  CodeFreqIn : Inport
  AddSub : xbsIndex_r4/AddSub  mode=Addition  use_carryin=off  use_carryout=off  en=off  latency=0  precision=User Defined  arith_type=Unsigned  n_bits=32  bin_pt=22  quantization=Truncate  overflow=Flag as error  use_behavioral_HDL=off  hw_selection=Fabric  pipelined=off  dbl_ovrd=off  block_type=addsub
  Convert : xbsIndex_r4/Convert  gui_display_data_type=Fixed-point  arith_type=Unsigned  n_bits=10  bin_pt=0  float_type=Single  exp_bits=8  fraction_bits=24  quantization=Truncate  overflow=Wrap  en=off  latency=1  pipeline=off  dbl_ovrd=off  block_type=convert
  Modulo : xbsIndex_r4/Constant  const=1023-2e-22  gui_display_data_type=Fixed-point  arith_type=Unsigned  n_bits=32  bin_pt=22  preci_type=Single  exp_width=8  frac_width=24  explicit_period=on  period=1/16367600  equ=P=C  opselect=C  inp2=PCIN>>17  opr=+  inp1=P  carry=CIN  dbl_ovrd=off  block_type=constant
  ModuloGen : xbsIndex_r4/AddSub  mode=Subtraction  use_carryin=off  use_carryout=off  en=off  latency=0  precision=User Defined  arith_type=Unsigned  n_bits=32  bin_pt=22  quantization=Truncate  overflow=Wrap  use_behavioral_HDL=off  hw_selection=Fabric  pipelined=off  dbl_ovrd=off  block_type=addsub
  Mux1 : xbsIndex_r4/Mux  inputs=2  en=off  latency=0  precision=Full  arith_type=Unsigned  n_bits=16  bin_pt=14  quantization=Truncate  overflow=Wrap  dbl_ovrd=off  block_type=mux
  ROM : xbsIndex_r4/ROM  depth=1023  initVector=[1,-1,-1,1,-1,1,1,-1,1,1,-1,-1,-1,1,-1,-1,-1,1,1,-1,1,1,-1,-1,-1,1,-1,1,-1,1,1,1,-1,-1,-1,1,1,1,1,-1,1,-1,1,-1,1,1,1,-1,1,1,1,1,1,-1,-1,1,1,-1,1,1,1,1,1,-1,1,-1,1,-1,-1,-1,1,1,1,1,1,-1,1,1,1,-1,-1,1,-1,-1,-1,1,-1,1,1,-1,-1,1,-1,-1,1,1,1,-1,1,-1,1,1,1,1,-1,1,1,-1,-1,1,-1,-1,1,-1,-1,-1,-1,1,1,-1,-1,-1,-1,-1,-1,-1,-1,1,1,1,-1,-1,-1,-1,-1,-1,1,1,1,-1,-1,1,1,1,1,-1,1,1,1,1,-1,1,-1,-1,1,-1,-1,1,1,-1,1,1,-1,1,1,1,-1,1,1,-1,-1,1,-1,1,1,-1,1,1,1,1,-1,-1,1,1,1,1,-1,1,1,1,-1,-1,1,-1,-1,1,1,-1,1,1,-1,1,1,-1,-1,1,1,1,-1,-1,-1,1,-1,-1,-1,-1,-1,-1,-1,1,-1,-1,1,-1,-1,1,-1,1,-1,-1,-1,1,1,1,1,1,1,1,1,-1,-1,-1,-1,1,1,1,-1,-1,1,-1,1,1,-1,1,1,-1,1,-1,-1,-1,1,1,1,-1,-1,1,1,1,-1,1,1,1,-1,1,-1,-1,-1,1,1,-1,1,1,1,-1,-1,-1,1,-1,1,-1,-1,-1,-1,-1,-1,1,-1,1,1,-1,1,-1,-1,-1,-1,1,-1,-1,1,1,-1,1,-1,1,1,1,1,-1,-1,-1,1,1,1,1,1,1,-1,-1,-1,1,-1,-1,1,1,-1,-1,1,1,-1,-1,-1,-1,-1,-1,-1,1,-1,1,1,1,1,1,1,1,1,1,-1,-1,1,1,-1,-1,-1,1,-1,1,1,-1,-1,1,-1,1,1,1,1,1,-1,-1,1,-1,-1,1,-1,-1,1,-1,1,-1,1,-1,-1,1,1,1,1,1,-1,1,-1,1,-1,1,1,-1,-1,1,-1,1,1,-1,1,-1,-1,1,-1,-1,1,1,-1,-1,-1,-1,-1,-1,-1,1,1,-1,-1,-1,-1,-1,-1,1,-1,1,1,1,-1,1,1,-1,1,-1,-1,-1,-1,1,-1,-1,-1,1,1,1,1,-1,1,1,-1,1,1,-1,1,-1,-1,-1,1,1,-1,1,1,-1,-1,-1,-1,1,1,1,-1,1,-1,-1,1,-1,-1,-1,-1,1,1,1,-1,-1,-1,-1,1,1,-1,-1,1,1,-1,-1,-1,1,-1,-1,-1,-1,1,-1,1,-1,-1,1,-1,-1,-1,-1,-1,1,-1,-1,1,1,-1,1,-1,-1,1,-1,1,-1,-1,-1,1,-1,1,1,-1,1,1,-1,1,-1,1,-1,1,-1,1,-1,1,-1,-1,-1,1,1,1,-1,1,-1,1,1,1,-1,1,1,1,-1,-1,-1,-1,1,-1,1,1,-1,-1,1,-1,1,-1,1,-1,1,1,1,1,1,1,1,1,1,-1,-1,-1,1,-1,-1,1,1,1,1,1,1,-1,-1,1,-1,-1,1,-1,-1,1,-1,-1,-1,-1,-1,-1,-1,1,1,-1,1,1,-1,1,1,1,-1,-1,-1,-1,1,-1,1,-1,1,1,1,1,-1,1,1,-1,1,1,1,1,1,-1,-1,-1,-1,1,-1,-1,1,1,-1,-1,1,1,1,-1,1,1,1,1,-1,-1,-1,1,1,1,1,1,-1,1,-1,1,-1,1,-1,-1,1,1,1,-1,1,-1,-1,1,1,1,-1,1,-1,-1,-1,-1,-1,1,1,1,-1,1,-1,-1,1,1,1,-1,-1,1,1,1,1,1,-1,1,-1,-1,-1,1,1,1,-1,1,1,1,1,-1,-1,-1,1,1,1,-1,-1,-1,1,-1,-1,1,-1,-1,-1,-1,1,-1,1,1,1,-1,1,1,1,-1,1,1,-1,-1,1,-1,-1,1,-1,-1,1,1,-1,-1,1,1,-1,-1,-1,-1,-1,-1,1,1,-1,1,1,-1,1,-1,-1,-1,1,1,1,-1,1,-1,1,1,1,-1,1,-1,1,-1,-1,-1,1,1,1,-1,-1,-1,-1,-1,-1,1,1,-1,1,-1,-1,-1,-1,1,1,1,-1,-1,-1,-1,1,-1,1,-1,1,-1,-1,-1,-1,-1,-1,1,1,1,1,1,1,-1,-1,1,1,-1,1,1,1,1,-1,1,1,-1,1,-1,1,-1,1,-1,1,-1,-1,1,-1,-1,-1,1,1,-1,-1,-1,-1,-1,-1,-1,-1,1,1,-1,-1,1,-1,-1,1,-1,1,-1,1,1,1,-1,1,-1,-1,1,1,1,1,1,-1,-1,1,-1,-1,1,1,-1,-1,1,1,-1,1,-1,-1,1,-1,1,-1,-1,-1,1,1,-1,1,-1,1,-1,1,-1,-1,1,1,1,1,-1,-1,-1,-1,-1,-1,1,1,1,1,1,-1,-1,1,-1,-1,-1,1,1,1,-1,1,-1,1,-1,1,-1,1,1,-1,-1,-1,1,-1,1,1,1,-1,-1,1,1,1,1,-1,1,-1,1,1,-1,1,-1,1,-1,-1,1,1,-1,1,-1,-1,-1,-1,-1,1,-1,-1,1,1,-1,1,-1,1,-1,-1,1,1,1,-1,-1,1,-1]  distributed_mem=Block RAM  rst=off  init_reg=0  en=off  latency=1  gui_display_data_type=Fixed-point  arith_type="Signed  (2's comp)"  n_bits=2  bin_pt=0  preci_type=Single  exp_width=8  frac_width=24  optimize=Area  use_rpm=on  dbl_ovrd=off  block_type=sprom
  Register : xbsIndex_r4/Register  init=0  rst=off  en=off  dbl_ovrd=off  block_type=register
  Relational : xbsIndex_r4/Relational  mode=a>=b  op_type=Bool  en=off  latency=0  dbl_ovrd=off  block_type=relational
  ROM Out : Outport
  Addr Out : Outport  Port=2
  EN Out : Outport  Port=3
  wires:
  Relational/1 -> EN Out/1, Mux1/1
  Convert/1 -> ROM/1, Addr Out/1
  ROM/1 -> ROM Out/1
  CodeFreqIn/1 -> AddSub/1
  Mux1/1 -> Register/1
  AddSub/1 -> ModuloGen/1, Relational/1, Mux1/2
  ModuloGen/1 -> Mux1/3
  Modulo/1 -> ModuloGen/2, Relational/2
  Register/1 -> Convert/1, AddSub/2
